simulink model "AEB_Test_module"  (R2017b)
settings: Solver=ode8  StartTime=0.0  StopTime=100.0  FixedStep=0.01  RelTol=1e-3
libraries: SimOneModule x3
settings Model: Creator=xuliang  LastModifiedBy=xuliang
settings DebuggingCC: ParameterPrecisionLossMsg=none

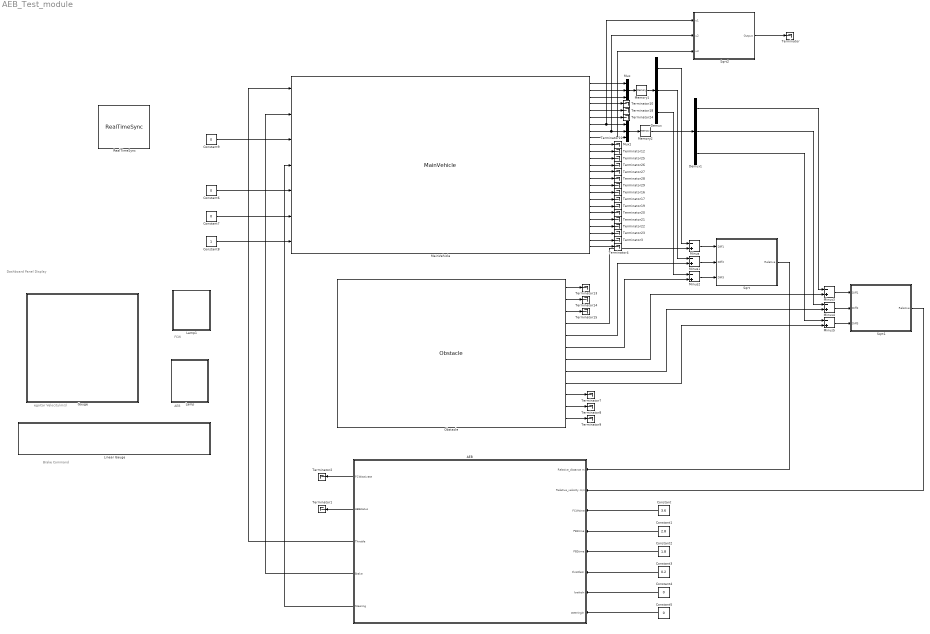
== system AEB_Test_module ==
  note: FCW
  note: egoCar Velocity(m/s)
  note: AEB
  note: Dashboard Panel Display
  note: Brake Command
  AEB : Subsystem  mask(AEB){}
      mask help: AEB block
  Constant : Constant  Value=3.6  OutDataTypeStr=single
  Constant1 : Constant  Value=2.8  OutDataTypeStr=single
  Constant2 : Constant  Value=1.8  OutDataTypeStr=single
  Constant3 : Constant  Value=0.2  OutDataTypeStr=single
  Constant4 : Constant  Value=0  OutDataTypeStr=single
  Constant5 : Constant  Value=0  OutDataTypeStr=single
  Constant6 : Constant  Value=0  OutDataTypeStr=boolean
  Constant7 : Constant  Value=0  OutDataTypeStr=boolean
  Constant8 : Constant  OutDataTypeStr=int32
  Constant9 : Constant  Value=0  OutDataTypeStr=int32
  Demux : Demux  Outputs=3
  Demux1 : Demux  Outputs=3
  Gauge : Subsystem  DialogController=hmiCreateDDGDialog  IsWebBlock=on  mask(MWDashboardBlock){webBlockId=47d9afb7-ca15-4b52-9b06-8f3727cd5279, webBlockType=circulargauge, ShowInLibBrowser=on, ShowInitialText=on, HMISrcModelName=AEB_Test_module}
      mask prompts: webBlockId "WebBlock Id"; webBlockType "WebBlock Type"; HMISrcModelName "Source Model"
      mask help: SimulinkHMI:dialogs:CircularGaugeDialogDesc
      mask Help: helpview([docroot '/mapfiles/simulink.map'], 'hmi_gauge')
      mask Display:
      | if strcmp(get_param(bdroot(gcb),'BlockDiagramType'), 'library')
      |     image([(matlabroot) '/toolbox/simulink/hmi/icons/CircularGauge.png']);
      | end
  Lamp : Subsystem  DialogController=hmiCreateDDGDialog  IsWebBlock=on  mask(MWDashboardBlock){webBlockId=ea335408-2001-4d64-815b-9b0ee8246115, webBlockType=lamp, ShowInLibBrowser=on, ShowInitialText=on, HMISrcModelName=AEB_Test_module}
      mask prompts: webBlockId "WebBlock Id"; webBlockType "WebBlock Type"; HMISrcModelName "Source Model"
      mask help: Display a color that reflects an input value.
      mask Help: helpview([docroot '/mapfiles/simulink.map'], 'hmi_lamp')
      mask Display:
      | if strcmp(get_param(bdroot(gcb),'BlockDiagramType'),'library')
      |  image([(matlabroot) '/toolbox/simulink/hmi/icons/Lamp.png'])
      | end
  Lamp1 : Subsystem  DialogController=hmiCreateDDGDialog  IsWebBlock=on  mask(MWDashboardBlock){webBlockId=ff899b74-b3e1-4288-b72d-9039b9796b1c, webBlockType=lamp, ShowInLibBrowser=on, ShowInitialText=on, HMISrcModelName=AEB_Test_module}
      mask prompts: webBlockId "WebBlock Id"; webBlockType "WebBlock Type"; HMISrcModelName "Source Model"
      mask help: Display a color that reflects an input value.
      mask Help: helpview([docroot '/mapfiles/simulink.map'], 'hmi_lamp')
      mask Display:
      | if strcmp(get_param(bdroot(gcb),'BlockDiagramType'),'library')
      |  image([(matlabroot) '/toolbox/simulink/hmi/icons/Lamp.png'])
      | end
  Linear Gauge : Subsystem  DialogController=hmiCreateDDGDialog  IsWebBlock=on  mask(MWDashboardBlock){webBlockId=739a4254-edef-4805-a255-418ead3e1f6d, webBlockType=lineargauge, ShowInLibBrowser=on, ShowInitialText=on, HMISrcModelName=AEB_Test_module}
      mask prompts: webBlockId "WebBlock Id"; webBlockType "WebBlock Type"; HMISrcModelName "Source Model"
      mask help: SimulinkHMI:dialogs:LinearGaugeDialogDesc
      mask Help: helpview([docroot '/mapfiles/simulink.map'], 'hmi_linear_gauge')
      mask Display:
      | if strcmp(get_param(bdroot(gcb),'BlockDiagramType'), 'library')
      |     image([(matlabroot) '/toolbox/simulink/hmi/icons/LinearGauge.png']);
      | end
  MainVehicle : SimOneModule/MainVehicle
  Memory1 : Memory
  Memory2 : Memory
  Minus{,1..5} (6 alike) : Sum  Inputs=-+
  Mux : Mux  Inputs=3
  Mux1 : Mux  Inputs=3
  Obstacle : SimOneModule/Obstacle  MaxObstacleNum=10  ObstacleId=1
  RealTimeSync : SimOneModule/RealTimeSync
  Sqrt : Subsystem  mask(Sqrt){}
      mask help: Square root of the sum of squared inputs
  Sqrt1 : Subsystem  mask(Sqrt){}
      mask help: Square root of the sum of squared inputs
  Sqrt2 : Subsystem  mask(Sqrt){}
      mask help: Square root of the sum of squared inputs
  Terminator{,1..4,7..29} (28 alike) : Terminator
  wires:
  Mux/1 -> Memory1/1
  Constant2/1 -> AEB/5(PB2time)
  Constant1/1 -> AEB/4(PB1time)
  Constant/1 -> AEB/3(FCWtime)
  AEB/1(FCWactivate) -> Terminator2/1
  AEB/2(AEBstatus) -> Terminator1/1
  Constant6/1 -> MainVehicle/5
  Constant7/1 -> MainVehicle/6
  Constant8/1 -> MainVehicle/7
  Constant3/1 -> AEB/6(throttleIn)
  Constant4/1 -> AEB/7(brakeIn)
  Constant5/1 -> AEB/8(steeringIn)
  AEB/5(Steering) -> MainVehicle/4
  AEB/3(Throttle) -> MainVehicle/1
  AEB/4(Brake) -> MainVehicle/2
  Obstacle/5 -> Minus1/2
  Demux/2 -> Minus1/1
  Obstacle/6 -> Minus2/2
  Obstacle/4 -> Minus/2
  Demux/1 -> Minus/1
  Demux/3 -> Minus2/1
  Minus1/1 -> Sqrt/2(Diff2)
  Minus/1 -> Sqrt/1(Diff1)
  Minus2/1 -> Sqrt/3(Diff3)
  Sqrt/1(Relative) -> AEB/1(Relative_distance m)
  Obstacle/8 -> Minus4/2
  Demux1/2 -> Minus4/1
  Obstacle/7 -> Minus3/2
  Demux1/3 -> Minus5/1
  Minus3/1 -> Sqrt1/1(Diff1)
  Minus4/1 -> Sqrt1/2(Diff2)
  Minus5/1 -> Sqrt1/3(Diff3)
  Demux1/1 -> Minus3/1
  Memory1/1 -> Demux/1
  Memory2/1 -> Demux1/1
  Obstacle/10 -> Terminator7/1
  MainVehicle/4 -> Terminator10/1
  MainVehicle/10 -> Terminator11/1
  MainVehicle/11 -> Terminator12/1
  Obstacle/1 -> Terminator13/1
  Obstacle/2 -> Terminator14/1
  MainVehicle/17 -> Terminator16/1
  MainVehicle/18 -> Terminator17/1
  MainVehicle/19 -> Terminator19/1
  MainVehicle/20 -> Terminator20/1
  MainVehicle/21 -> Terminator21/1
  MainVehicle/22 -> Terminator22/1
  MainVehicle/23 -> Terminator23/1
  MainVehicle/1 -> Mux/1
  MainVehicle/2 -> Mux/2
  MainVehicle/3 -> Mux/3
  MainVehicle/5 -> Terminator18/1
  MainVehicle/6 -> Terminator24/1
  MainVehicle/7 -> Sqrt2/1(u1), Mux1/1
  MainVehicle/8 -> Mux1/2, Sqrt2/2(u2)
  MainVehicle/9 -> Mux1/3, Sqrt2/3(u3)
  Mux1/1 -> Memory2/1
  MainVehicle/12 -> Terminator25/1
  MainVehicle/13 -> Terminator26/1
  MainVehicle/14 -> Terminator27/1
  MainVehicle/15 -> Terminator28/1
  MainVehicle/16 -> Terminator29/1
  Obstacle/3 -> Terminator15/1
  Obstacle/12 -> Terminator9/1
  Obstacle/11 -> Terminator8/1
  Obstacle/9 -> Minus5/2
  Sqrt2/1(Output) -> Terminator/1
  Sqrt1/1(Relative) -> AEB/2(Relative_velocity m/s)
  MainVehicle/24 -> Terminator3/1
  MainVehicle/25 -> Terminator4/1
  Constant9/1 -> MainVehicle/3

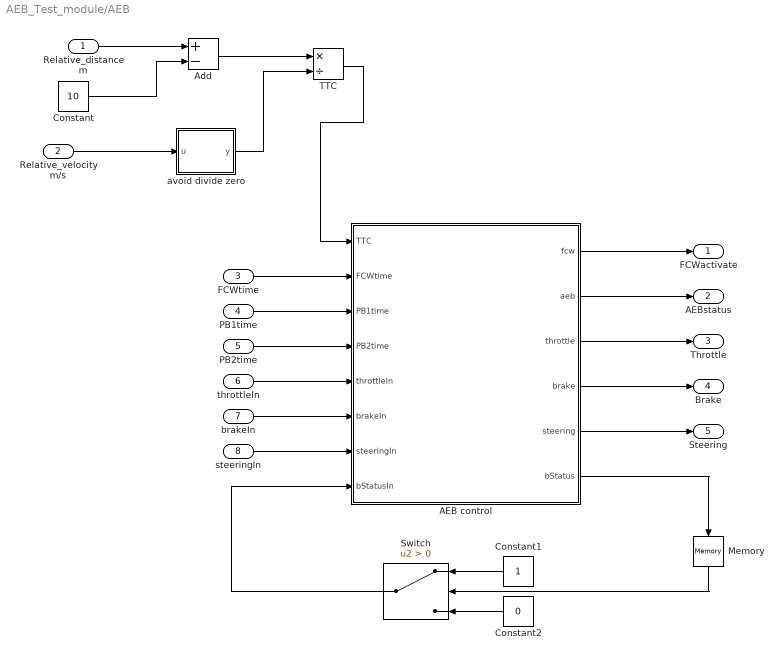
== system AEB_Test_module/AEB ==
  Relative_distance m : Inport
  Relative_velocity m/s : Inport  Port=2
  FCWtime : Inport  Port=3
  PB1time : Inport  Port=4
  PB2time : Inport  Port=5
  throttleIn : Inport  Port=6
  brakeIn : Inport  Port=7
  steeringIn : Inport  Port=8
  AEB control : MATLAB Function  TreatAsAtomicUnit=on
  Add : Sum  Inputs=+-
  Constant : Constant  Value=10  OutDataTypeStr=single
  Constant1 : Constant  OutDataTypeStr=double
  Constant2 : Constant  Value=0  OutDataTypeStr=double
  Memory : Memory
  Switch : Switch  Criteria=u2 > Threshold
  TTC : Product  Inputs=*/
  avoid divide zero : MATLAB Function  TreatAsAtomicUnit=on
  FCWactivate : Outport
  AEBstatus : Outport  Port=2
  Throttle : Outport  Port=3
  Brake : Outport  Port=4
  Steering : Outport  Port=5
  wires:
  Relative_distance m/1 -> Add/1
  Constant/1 -> Add/2
  Relative_velocity m/s/1 -> avoid divide zero/1(u)
  Add/1 -> TTC/1
  avoid divide zero/1(y) -> TTC/2
  TTC/1 -> AEB control/1(TTC)
  PB2time/1 -> AEB control/4(PB2time)
  PB1time/1 -> AEB control/3(PB1time)
  AEB control/2(aeb) -> AEBstatus/1
  FCWtime/1 -> AEB control/2(FCWtime)
  AEB control/1(fcw) -> FCWactivate/1
  AEB control/4(brake) -> Brake/1
  throttleIn/1 -> AEB control/5(throttleIn)
  brakeIn/1 -> AEB control/6(brakeIn)
  steeringIn/1 -> AEB control/7(steeringIn)
  Switch/1 -> AEB control/8(bStatusIn)
  AEB control/3(throttle) -> Throttle/1
  AEB control/6(bStatus) -> Memory/1
  AEB control/5(steering) -> Steering/1
  Constant1/1 -> Switch/1
  Constant2/1 -> Switch/3
  Memory/1 -> Switch/2

== system AEB_Test_module/Gauge ==

== system AEB_Test_module/Lamp ==

== system AEB_Test_module/Lamp1 ==

== system AEB_Test_module/Linear Gauge ==

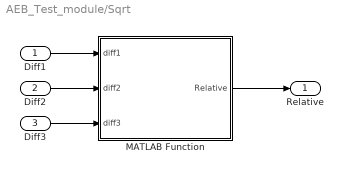
== system AEB_Test_module/Sqrt ==
  Diff1 : Inport
  Diff2 : Inport  Port=2
  Diff3 : Inport  Port=3
  MATLAB Function : MATLAB Function  TreatAsAtomicUnit=on
  Relative : Outport
  wires:
  Diff1/1 -> MATLAB Function/1(diff1)
  MATLAB Function/1(Relative) -> Relative/1
  Diff2/1 -> MATLAB Function/2(diff2)
  Diff3/1 -> MATLAB Function/3(diff3)

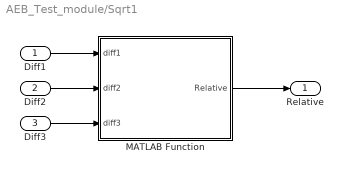
== system AEB_Test_module/Sqrt1 ==
  Diff1 : Inport
  Diff2 : Inport  Port=2
  Diff3 : Inport  Port=3
  MATLAB Function : MATLAB Function  TreatAsAtomicUnit=on
  Relative : Outport
  wires:
  Diff1/1 -> MATLAB Function/1(diff1)
  MATLAB Function/1(Relative) -> Relative/1
  Diff2/1 -> MATLAB Function/2(diff2)
  Diff3/1 -> MATLAB Function/3(diff3)

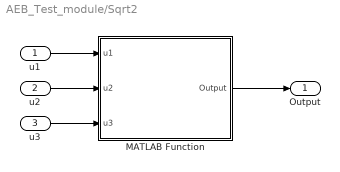
== system AEB_Test_module/Sqrt2 ==
  u1 : Inport
  u2 : Inport  Port=2
  u3 : Inport  Port=3
  MATLAB Function : MATLAB Function  TreatAsAtomicUnit=on
  Output : Outport
  wires:
  u1/1 -> MATLAB Function/1(u1)
  MATLAB Function/1(Output) -> Output/1
  u2/1 -> MATLAB Function/2(u2)
  u3/1 -> MATLAB Function/3(u3)

== matlab function AEB_Test_module/AEB/AEB control ==
  data: fcw output; aeb output; throttle output; brake output; TTC input; FCWtime input; PB1time input; PB2time input; throttleIn input; brakeIn input; steeringIn input; bStatusIn input; steering output; bStatus output
function [fcw,aeb,throttle,brake,steering,bStatus] = fcn(TTC,FCWtime,PB1time,PB2time,throttleIn, brakeIn,steeringIn,bStatusIn)
throttle = throttleIn;
brake = brakeIn;
steering = steeringIn;
bStatus = bStatusIn;
if(bStatusIn > 0)
    throttle = single(0.0);
end
if(abs(TTC) >= FCWtime || TTC>=0)
    aeb = 0;
    fcw = 0;
else
    aeb = 0;
    fcw = 1;
    bStatus = 1;
    brake = single(0.1);
    if(abs(TTC) < PB2time)
       aeb = 2;
       brake = single(0.4);
    end
    if(abs(TTC) < PB1time)
       aeb = 1;
       brake = single(0.3);
    end
end

== matlab function AEB_Test_module/AEB/avoid divide zero ==
  data: u input; y output
function y  = fcn(u)
if (abs(u)<0.001)
    y = 0.001 * sign(u);
    if(u == 0)
        y = single(0.001);
    end
else
    y = u;
end

== matlab function AEB_Test_module/Sqrt/MATLAB Function ==
  data: diff1 input; Relative output; diff2 input; diff3 input
function Relative = fcn(diff1,diff2,diff3)

Relative = sqrt(diff1 * diff1 + diff2 * diff2 + diff3 * diff3);

== matlab function AEB_Test_module/Sqrt1/MATLAB Function ==
  data: diff1 input; Relative output; diff2 input; diff3 input
function Relative = fcn(diff1,diff2,diff3)

Relative = sqrt(diff1 * diff1 + diff2 * diff2 + diff3 * diff3) * sign(diff1);

== matlab function AEB_Test_module/Sqrt2/MATLAB Function ==
  data: u1 input; Output output; u2 input; u3 input
function Output = fcn(u1,u2,u3)

Output = sqrt(u1 * u1 + u2 * u2 + u3 * u3);
